simulink model "Lab1A"  (R2020a)
settings: Solver=VariableStepAuto  StartTime=0.0  StopTime=0.2  RelTol=1e-3
values from neighbouring files (symbols this model uses):
  E = 10    [LAB2.m]
  L = 0.05    [LAB2.m]
  R = 2    [LAB2.m]
settings Model: Creator=98all  LastModifiedBy=98all
settings DataIOCC: ReturnWorkspaceOutputs=off  TimeSaveName=tdc

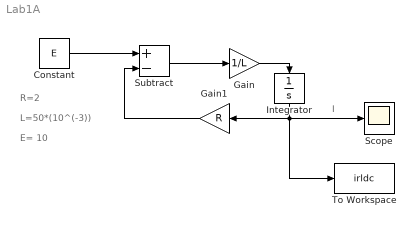
== system Lab1A ==
  note: I
  note: E= 10
  note: L=50*(10^(-3))
  note: R=2
  Constant : Constant  Value=E
  Gain : Gain  Gain=1/L
  Gain1 : Gain  Gain=R
  Integrator : Integrator
  Scope : Scope
  Subtract : Sum  Inputs=+-
  To Workspace : ToWorkspace  VariableName=irldc  SampleTime=-1
  wires:
  Constant/1 -> Subtract/1
  Subtract/1 -> Gain/1
  Gain/1 -> Integrator/1
  Integrator/1 -> To Workspace/1, Scope/1, Gain1/1
  Gain1/1 -> Subtract/2
